simulink model "Ex3_3_a_sim"  (R2017b)
settings: Solver=ode45  StartTime=0.0  StopTime=0.2  RelTol=1e-3  EnableMultiTasking=on
values from neighbouring files (symbols this model uses):
  K_e = 5e-2    (= 0.05)    [Ex3_3_a.m]    (also in Ex3_3_x2_StateSpace.m)
  K_t = 5e-2    (= 0.05)    [Ex3_3_a.m]    (also in Ex3_3_x2_StateSpace.m)
settings Model: Creator=Shin  LastModifiedBy=minakata
settings DataIOCC: LimitDataPoints=on  SaveFormat=Array
settings OptimizationCC: LifeSpan=inf
settings DebuggingCC: SolverPrmCheckMsg=warning  SFUnexpectedBacktrackingDiag=warning  SFNoUnconditionalDefaultTransitionDiag=warning  SFExecutionAtInitializationDiag=none
settings HardwareCC: ProdBitPerPointer=32  ProdBitPerSizeT=32  ProdBitPerPtrDiffT=32  ProdLargestAtomicFloat=None  ProdIntDivRoundTo=Undefined  ProdEndianess=Unspecified  ProdWordSize=32  ProdHWDeviceType=32-bit Generic
settings ModelReferenceCC: PropagateSignalLabelsOutOfModel=off
settings CodeAppCC: StateflowObjectComments=on
settings GRTTargetCC: TargetLangStandard=C89/C90 (ANSI)  GeneratePreprocessorConditionals=Disable all
settings ConfigComp: CovMetricSettings=dw  CovHtmlReporting=on  CovSaveCumulativeToWorkspaceVar=on  CovSaveSingleToWorkspaceVar=on  CovExternalEMLEnable=off  CovSFcnEnable=off

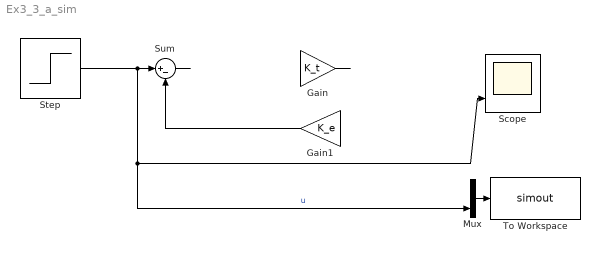
== system Ex3_3_a_sim ==
  Gain : Gain  Gain=K_t
  Gain1 : Gain  Gain=K_e
  Mux : Mux  Inputs=2
  Scope : Scope  NumInputPorts=2
  Step : Step  Time=0.01  SampleTime=0
  Sum : Sum  Inputs=|+-
  To Workspace : ToWorkspace  VariableName=simout  SaveFormat=Timeseries  SampleTime=-1
  wires:
  Step/1 -> Sum/1, Mux/2, Scope/2  "u"
  Mux/1 -> To Workspace/1
  ? -> Gain/1
  Sum/1 -> ?
  Gain/1 -> ?
  Gain1/1 -> Sum/2
  ? -> Scope/1, Gain1/1, Mux/1
